simulink model "dcmotorsys"  (R2016a)
settings: Solver=VariableStepAuto  StartTime=0.0  StopTime=10.0  RelTol=1e-3
values from neighbouring files (symbols this model uses):
  Bm = 0.02    [dcmotorscript.m]
  Jm = 6.8*10^(-4)    (= 0.00068)    [dcmotorscript.m]
  Kb = 0.8598    [dcmotorscript.m]
  Ki = 0.7    [dcmotorscript.m]
  La = 5.8*10^(-3)    (= 0.0058)    [dcmotorscript.m]
  Ra = 0.8    [dcmotorscript.m]
libraries: simulink x1
settings Model: Creator=Mohammed Bitar  LastModifiedBy=Mohammed Bitar

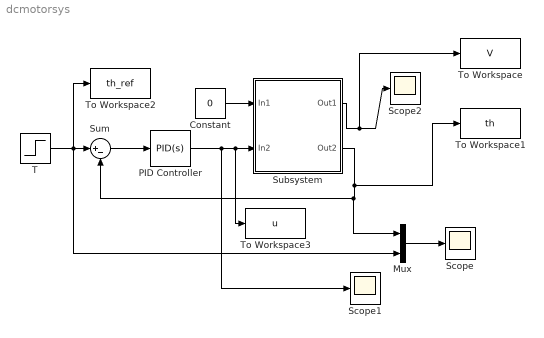
== system dcmotorsys ==
  Constant : Constant  Value=0
  Mux : Mux  Inputs=2
  PID Controller : simulink/Continuous/PID Controller  Controller=PID  TimeDomain=Continuous-time  SampleTime=-1  IntegratorMethod=Forward Euler  FilterMethod=Forward Euler  Form=Parallel  UseFilter=on  ControllerParametersSource=internal  P=45.8180732540142  I=475.189462987433  D=-0.153685385517573  N=298.12901922789  InitialConditionSource=internal  InitialConditionForIntegrator=0  InitialConditionForFilter=0  ExternalReset=none  LimitOutput=off  UpperSaturationLimit=inf  LowerSaturationLimit=-inf  LinearizeAsGain=on  AntiWindupMode=none  Kb=1  TrackingMode=off  Kt=1  PParamMin=[]  PParamMax=[]  IParamMin=[]  IParamMax=[]  DParamMin=[]  DParamMax=[]  NParamMin=[]  NParamMax=[]  KbParamMin=[]  KbParamMax=[]  KtParamMin=[]  KtParamMax=[]  POutMin=[]  POutMax=[]  IOutMin=[]  IOutMax=[]  DOutMin=[]  DOutMax=[]  NOutMin=[]  NOutMax=[]  KbOutMin=[]  KbOutMax=[]  KtOutMin=[]  KtOutMax=[]  IntegratorOutMin=[]  IntegratorOutMax=[]  FilterOutMin=[]  FilterOutMax=[]  SumOutMin=[]  SumOutMax=[]  SumI1OutMin=[]  SumI1OutMax=[]  SumI2OutMin=[]  SumI2OutMax=[]  SumI3OutMin=[]  SumI3OutMax=[]  SumDOutMin=[]  SumDOutMax=[]  SaturationOutMin=[]  SaturationOutMax=[]  IntegratorContinuousStateAttributes=''  IntegratorStateMustResolveToSignalObject=off  IntegratorRTWStateStorageClass=Auto  FilterContinuousStateAttributes=''  FilterStateMustResolveToSignalObject=off  FilterRTWStateStorageClass=Auto  DifferentiatorICPrevScaledInput=0  DifferentiatorOutMin=[]  DifferentiatorOutMax=[]
  Scope : Scope
  Scope1 : Scope
  Scope2 : Scope
  Subsystem : Subsystem
      mask Display:
      | color('red')
      | port_label('input',1,'T_L')
      | port_label('input',2,'Ref')
      | color('blue')
      | port_label('output',1,'v')
      | port_label('output',2,'th')
  Sum : Sum  Inputs=|+-
  T : Step  SampleTime=0
  To Workspace : ToWorkspace  VariableName=V  SampleTime=0.01
  To Workspace1 : ToWorkspace  VariableName=th  SampleTime=0.01
  To Workspace2 : ToWorkspace  VariableName=th_ref  SampleTime=0.01
  To Workspace3 : ToWorkspace  VariableName=u  SampleTime=0.01
  wires:
  Mux/1 -> Scope/1
  Constant/1 -> Subsystem/1(In1)
  PID Controller/1 -> Scope1/1, To Workspace3/1, Subsystem/2(In2)
  Sum/1 -> PID Controller/1
  Subsystem/1(Out1) -> To Workspace/1, Scope2/1
  T/1 -> To Workspace2/1, Mux/2, Sum/1
  Subsystem/2(Out2) -> To Workspace1/1, Mux/1, Sum/2

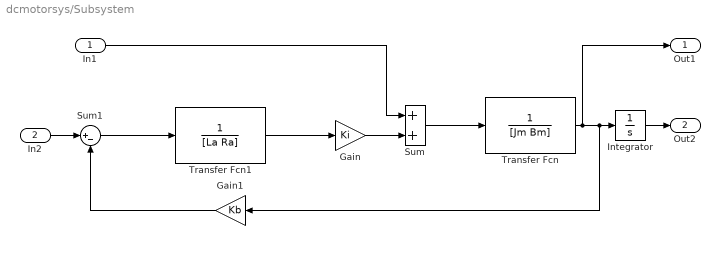
== system dcmotorsys/Subsystem ==
  In1 : Inport
  In2 : Inport  Port=2
  Gain : Gain  Gain=Ki
  Gain1 : Gain  Gain=Kb
  Integrator : Integrator
  Sum : Sum
  Sum1 : Sum  Inputs=|+-
  Transfer Fcn : TransferFcn  Denominator=[Jm Bm]
  Transfer Fcn1 : TransferFcn  Denominator=[La Ra]
  Out1 : Outport
  Out2 : Outport  Port=2
  wires:
  Gain1/1 -> Sum1/2
  Sum1/1 -> Transfer Fcn1/1
  Transfer Fcn1/1 -> Gain/1
  Gain/1 -> Sum/2
  In1/1 -> Sum/1
  Sum/1 -> Transfer Fcn/1
  In2/1 -> Sum1/1
  Transfer Fcn/1 -> Gain1/1, Integrator/1, Out1/1
  Integrator/1 -> Out2/1
